simulink model "PendulumWithDrag"  (R2022a)
settings: Solver=VariableStepAuto  StartTime=0.0  StopTime=10.0  RelTol=1e-3
model workspace (MAT data in the model file):
  A = 0.01
  L = 1
  M = 1
undefined symbols (not defined in the file): g, rho
settings Model: Creator=Adam Ghatta  LastModifiedBy=Adam Ghatta

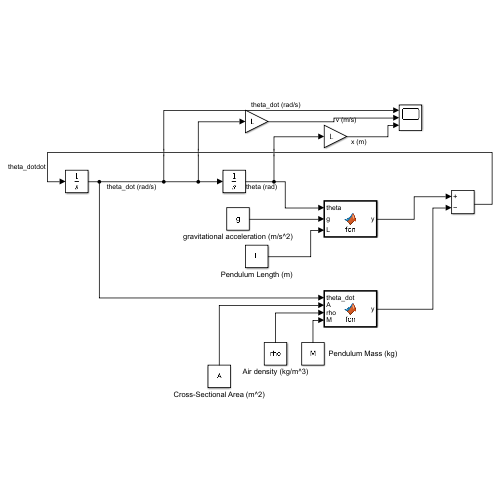
[thumbnail: Simulink's stored preview of the top-level diagram]
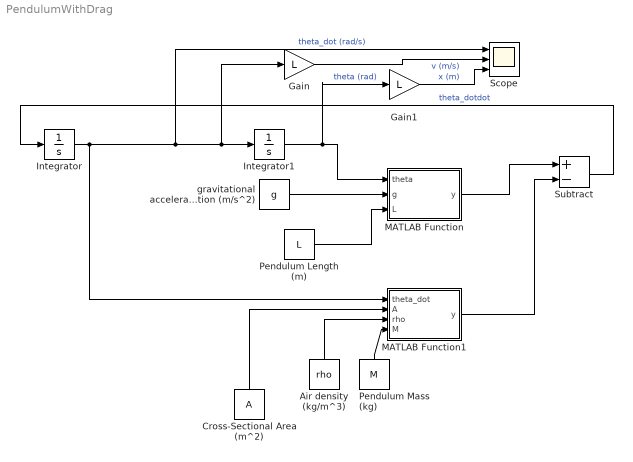
== system PendulumWithDrag ==
  Air density (kg/m^3) : Constant  Value=rho
  Cross-Sectional Area (m^2) : Constant  Value=A
  Gain : Gain  Gain=L
  Gain1 : Gain  Gain=L
  Integrator : Integrator
  Integrator1 : Integrator  InitialCondition=.14
  MATLAB Function : MATLAB Function  TreatAsAtomicUnit=on
  MATLAB Function1 : MATLAB Function  TreatAsAtomicUnit=on
  Pendulum Length (m) : Constant  Value=L
  Pendulum Mass (kg) : Constant  Value=M
  Scope : Scope  NumInputPorts=3
  Subtract : Sum  Inputs=+-
  gravitational acceleration (m/s^2) : Constant  Value=g
  wires:
  Integrator/1 -> MATLAB Function1/1(theta_dot), Scope/1, Gain/1, Integrator1/1  "theta_dot (rad/s)"
  Subtract/1 -> Integrator/1  "theta_dotdot"
  Integrator1/1 -> Gain1/1, MATLAB Function/1(theta)  "theta (rad)"
  gravitational acceleration (m/s^2)/1 -> MATLAB Function/2(g)
  Pendulum Length (m)/1 -> MATLAB Function/3(L)
  MATLAB Function/1(y) -> Subtract/1
  Cross-Sectional Area (m^2)/1 -> MATLAB Function1/2(A)
  Air density (kg/m^3)/1 -> MATLAB Function1/3(rho)
  Pendulum Mass (kg)/1 -> MATLAB Function1/4(M)
  MATLAB Function1/1(y) -> Subtract/2
  Gain/1 -> Scope/2  "v (m/s)"
  Gain1/1 -> Scope/3  "x (m)"

== matlab function PendulumWithDrag/MATLAB Function1 ==
  data: theta_dot input; y output; A input; rho input; M input
function y = fcn(theta_dot, A, rho, M)

y = (0.5 * rho * A* theta_dot)/(M);

== matlab function PendulumWithDrag/MATLAB Function ==
  data: theta input; y output; g input; L input
function y = fcn(theta, g, L)

y = (g / L) * sin(theta);
